simulink model "LoadLevel2_VF"  (R2023b)
settings: Solver=VariableStepAuto  StartTime=0.0  StopTime=250  RelTol=1e-3
undefined symbols (not defined in the file): a, Ac, Bc, Cc, D1, Dc, Delta, find_system, Fnom, gcbh, I21_init_imag, I21_init_real, Ibase1, Ibase2, Iw1A_init_mag, Iw1A_init_pha, Iw1B_init_mag, Iw1B_init_pha, Iw1C_init_mag, Iw1C_init_pha, Iw2A_init_mag, Iw2A_init_pha, Iw2B_init_mag, Iw2B_init_pha, Iw2C_init_mag, Iw2C_init_pha, j, kr, ks, Nmax, Pnom, psi, RegulatorDeadBand, RegulatorDelay, RegulatorVref, sps_rtmsupport, Vnom1, Vnom2, w, Z1pu, Z2pu, Ztpu
libraries: spsThreePhaseVIMeasurementLib x15, spsThreePhasePISectionLineLib x14, spsThreePhaseParallelRLCLoadLib x11, spsControlledCurrentSourceLib x6, spsThreePhaseTransformerTwoWindingsLib x5, spsThreePhaseBreakerLib x2, spsExcitationSystemLib x2, spsHydraulicTurbineandGovernorLib x2, spsSynchronousMachinepuStandardLib x2, spsThreePhaseSeriesRLCBranchLib x2, spsGroundLib x2, spsSequenceAnalyzerPhasorLib x1
(part 3 of 3)

== system LoadLevel2_VF/Three-Phase OLTC Regulating Transformer (Phasor Type)2/Voltage regulator/On//Off Delay/OFF Delay/Edge Detector ==
  note: Edge or Slope Detector
  In : Inport
  Constant1 : Constant  Value=model
  Demux : Demux  Outputs=2
      settings: DisplayOption=none
  Logical Operator1 : Logic  Operator=OR
  Memory : Memory  InitialCondition=ic  LinearizeAsDelay=on
  Multiport Switch : MultiPortSwitch  InputSameDT=off
  NEGATIVE Edge : Subsystem  TreatAsAtomicUnit=on
  POSITIVE Edge : Subsystem  TreatAsAtomicUnit=on
  either edge : Constant  Value=[1 1]
  neg. edge : Constant  Value=[0 1]
  pos. edge : Constant  Value=[1 0]
  Out : Outport  VectorParamsAs1DForOutWhenUnconnected=off
  wires:
  Logical Operator1/1 -> Out/1
  NEGATIVE Edge/1(OUT) -> Logical Operator1/2
  POSITIVE Edge/1(OUT) -> Logical Operator1/1
  Memory/1 -> POSITIVE Edge/2(IN previous), NEGATIVE Edge/2(IN previous)
  In/1 -> POSITIVE Edge/1(IN), NEGATIVE Edge/1(IN), Memory/1
  pos. edge/1 -> Multiport Switch/2
  neg. edge/1 -> Multiport Switch/3
  Constant1/1 -> Multiport Switch/1
  Multiport Switch/1 -> Demux/1
  Demux/1 -> POSITIVE Edge/Enable
  Demux/2 -> NEGATIVE Edge/Enable
  either edge/1 -> Multiport Switch/4

== system LoadLevel2_VF/Three-Phase OLTC Regulating Transformer (Phasor Type)2/Voltage regulator/On//Off Delay/OFF Delay/Sample & Hold ==
  note: Silvano Casoria
      | Power System Simulation Laboratory
      | IREQ, Hydro-Quebc
  note: Sample and Hold
  In : Inport
  S : Inport  Port=2
  IC=ic : Memory  InitialCondition=ic  InheritSampleTime=on
  Switch : Switch  Threshold=0.5
  "   " : Outport  InitialOutput=0  VectorParamsAs1DForOutWhenUnconnected=off
  wires:
  S/1 -> Switch/2
  In/1 -> Switch/1
  IC=ic/1 -> Switch/3
  Switch/1 -> IC=ic/1, "   "/1

== system LoadLevel2_VF/Three-Phase OLTC Regulating Transformer (Phasor Type)2/Voltage regulator/On//Off Delay/ON Delay/Edge Detector ==
  note: Edge or Slope Detector
  In : Inport
  Constant1 : Constant  Value=model
  Demux : Demux  Outputs=2
      settings: DisplayOption=none
  Logical Operator1 : Logic  Operator=OR
  Memory : Memory  InitialCondition=ic  LinearizeAsDelay=on
  Multiport Switch : MultiPortSwitch  InputSameDT=off
  NEGATIVE Edge : Subsystem  TreatAsAtomicUnit=on
  POSITIVE Edge : Subsystem  TreatAsAtomicUnit=on
  either edge : Constant  Value=[1 1]
  neg. edge : Constant  Value=[0 1]
  pos. edge : Constant  Value=[1 0]
  Out : Outport  VectorParamsAs1DForOutWhenUnconnected=off
  wires:
  Logical Operator1/1 -> Out/1
  NEGATIVE Edge/1(OUT) -> Logical Operator1/2
  POSITIVE Edge/1(OUT) -> Logical Operator1/1
  Memory/1 -> POSITIVE Edge/2(IN previous), NEGATIVE Edge/2(IN previous)
  In/1 -> POSITIVE Edge/1(IN), NEGATIVE Edge/1(IN), Memory/1
  pos. edge/1 -> Multiport Switch/2
  neg. edge/1 -> Multiport Switch/3
  Constant1/1 -> Multiport Switch/1
  Multiport Switch/1 -> Demux/1
  Demux/1 -> POSITIVE Edge/Enable
  Demux/2 -> NEGATIVE Edge/Enable
  either edge/1 -> Multiport Switch/4

== system LoadLevel2_VF/Three-Phase OLTC Regulating Transformer (Phasor Type)2/Voltage regulator/On//Off Delay/ON Delay/Sample & Hold ==
  note: Silvano Casoria
      | Power System Simulation Laboratory
      | IREQ, Hydro-Quebc
  note: Sample and Hold
  In : Inport
  S : Inport  Port=2
  IC=ic : Memory  InitialCondition=ic  InheritSampleTime=on
  Switch : Switch  Threshold=0.5
  "   " : Outport  InitialOutput=0  VectorParamsAs1DForOutWhenUnconnected=off
  wires:
  S/1 -> Switch/2
  In/1 -> Switch/1
  IC=ic/1 -> Switch/3
  Switch/1 -> IC=ic/1, "   "/1

== system LoadLevel2_VF/Three-Phase OLTC Regulating Transformer (Phasor Type)2/Voltage regulator/On//Off Delay1/OFF Delay/Edge Detector ==
  note: Edge or Slope Detector
  In : Inport
  Constant1 : Constant  Value=model
  Demux : Demux  Outputs=2
      settings: DisplayOption=none
  Logical Operator1 : Logic  Operator=OR
  Memory : Memory  InitialCondition=ic  LinearizeAsDelay=on
  Multiport Switch : MultiPortSwitch  InputSameDT=off
  NEGATIVE Edge : Subsystem  TreatAsAtomicUnit=on
  POSITIVE Edge : Subsystem  TreatAsAtomicUnit=on
  either edge : Constant  Value=[1 1]
  neg. edge : Constant  Value=[0 1]
  pos. edge : Constant  Value=[1 0]
  Out : Outport  VectorParamsAs1DForOutWhenUnconnected=off
  wires:
  Logical Operator1/1 -> Out/1
  NEGATIVE Edge/1(OUT) -> Logical Operator1/2
  POSITIVE Edge/1(OUT) -> Logical Operator1/1
  Memory/1 -> POSITIVE Edge/2(IN previous), NEGATIVE Edge/2(IN previous)
  In/1 -> POSITIVE Edge/1(IN), NEGATIVE Edge/1(IN), Memory/1
  pos. edge/1 -> Multiport Switch/2
  neg. edge/1 -> Multiport Switch/3
  Constant1/1 -> Multiport Switch/1
  Multiport Switch/1 -> Demux/1
  Demux/1 -> POSITIVE Edge/Enable
  Demux/2 -> NEGATIVE Edge/Enable
  either edge/1 -> Multiport Switch/4

== system LoadLevel2_VF/Three-Phase OLTC Regulating Transformer (Phasor Type)2/Voltage regulator/On//Off Delay1/OFF Delay/Sample & Hold ==
  note: Silvano Casoria
      | Power System Simulation Laboratory
      | IREQ, Hydro-Quebc
  note: Sample and Hold
  In : Inport
  S : Inport  Port=2
  IC=ic : Memory  InitialCondition=ic  InheritSampleTime=on
  Switch : Switch  Threshold=0.5
  "   " : Outport  InitialOutput=0  VectorParamsAs1DForOutWhenUnconnected=off
  wires:
  S/1 -> Switch/2
  In/1 -> Switch/1
  IC=ic/1 -> Switch/3
  Switch/1 -> IC=ic/1, "   "/1

== system LoadLevel2_VF/Three-Phase OLTC Regulating Transformer (Phasor Type)2/Voltage regulator/On//Off Delay1/ON Delay/Edge Detector ==
  note: Edge or Slope Detector
  In : Inport
  Constant1 : Constant  Value=model
  Demux : Demux  Outputs=2
      settings: DisplayOption=none
  Logical Operator1 : Logic  Operator=OR
  Memory : Memory  InitialCondition=ic  LinearizeAsDelay=on
  Multiport Switch : MultiPortSwitch  InputSameDT=off
  NEGATIVE Edge : Subsystem  TreatAsAtomicUnit=on
  POSITIVE Edge : Subsystem  TreatAsAtomicUnit=on
  either edge : Constant  Value=[1 1]
  neg. edge : Constant  Value=[0 1]
  pos. edge : Constant  Value=[1 0]
  Out : Outport  VectorParamsAs1DForOutWhenUnconnected=off
  wires:
  Logical Operator1/1 -> Out/1
  NEGATIVE Edge/1(OUT) -> Logical Operator1/2
  POSITIVE Edge/1(OUT) -> Logical Operator1/1
  Memory/1 -> POSITIVE Edge/2(IN previous), NEGATIVE Edge/2(IN previous)
  In/1 -> POSITIVE Edge/1(IN), NEGATIVE Edge/1(IN), Memory/1
  pos. edge/1 -> Multiport Switch/2
  neg. edge/1 -> Multiport Switch/3
  Constant1/1 -> Multiport Switch/1
  Multiport Switch/1 -> Demux/1
  Demux/1 -> POSITIVE Edge/Enable
  Demux/2 -> NEGATIVE Edge/Enable
  either edge/1 -> Multiport Switch/4

== system LoadLevel2_VF/Three-Phase OLTC Regulating Transformer (Phasor Type)2/Voltage regulator/On//Off Delay1/ON Delay/Sample & Hold ==
  note: Silvano Casoria
      | Power System Simulation Laboratory
      | IREQ, Hydro-Quebc
  note: Sample and Hold
  In : Inport
  S : Inport  Port=2
  IC=ic : Memory  InitialCondition=ic  InheritSampleTime=on
  Switch : Switch  Threshold=0.5
  "   " : Outport  InitialOutput=0  VectorParamsAs1DForOutWhenUnconnected=off
  wires:
  S/1 -> Switch/2
  In/1 -> Switch/1
  IC=ic/1 -> Switch/3
  Switch/1 -> IC=ic/1, "   "/1

== system LoadLevel2_VF/Three-Phase OLTC Regulating Transformer (Phasor Type)2/Voltage regulator/On//Off Delay/OFF Delay/Edge Detector/NEGATIVE Edge ==
  IN : Inport
  IN previous : Inport  Port=2
  Enable : EnablePort  PropagateVarSize=During execution
  Relational Operator1 : RelationalOperator  Operator=>
  OUT : Outport  VectorParamsAs1DForOutWhenUnconnected=off
  wires:
  Relational Operator1/1 -> OUT/1
  IN previous/1 -> Relational Operator1/1
  IN/1 -> Relational Operator1/2

== system LoadLevel2_VF/Three-Phase OLTC Regulating Transformer (Phasor Type)2/Voltage regulator/On//Off Delay/OFF Delay/Edge Detector/POSITIVE Edge ==
  IN : Inport
  IN previous : Inport  Port=2
  Enable : EnablePort  PropagateVarSize=During execution
  Relational Operator1 : RelationalOperator  Operator=>
  OUT : Outport  VectorParamsAs1DForOutWhenUnconnected=off
  wires:
  Relational Operator1/1 -> OUT/1
  IN previous/1 -> Relational Operator1/2
  IN/1 -> Relational Operator1/1

== system LoadLevel2_VF/Three-Phase OLTC Regulating Transformer (Phasor Type)2/Voltage regulator/On//Off Delay/ON Delay/Edge Detector/NEGATIVE Edge ==
  IN : Inport
  IN previous : Inport  Port=2
  Enable : EnablePort  PropagateVarSize=During execution
  Relational Operator1 : RelationalOperator  Operator=>
  OUT : Outport  VectorParamsAs1DForOutWhenUnconnected=off
  wires:
  Relational Operator1/1 -> OUT/1
  IN previous/1 -> Relational Operator1/1
  IN/1 -> Relational Operator1/2

== system LoadLevel2_VF/Three-Phase OLTC Regulating Transformer (Phasor Type)2/Voltage regulator/On//Off Delay/ON Delay/Edge Detector/POSITIVE Edge ==
  IN : Inport
  IN previous : Inport  Port=2
  Enable : EnablePort  PropagateVarSize=During execution
  Relational Operator1 : RelationalOperator  Operator=>
  OUT : Outport  VectorParamsAs1DForOutWhenUnconnected=off
  wires:
  Relational Operator1/1 -> OUT/1
  IN previous/1 -> Relational Operator1/2
  IN/1 -> Relational Operator1/1

== system LoadLevel2_VF/Three-Phase OLTC Regulating Transformer (Phasor Type)2/Voltage regulator/On//Off Delay1/OFF Delay/Edge Detector/NEGATIVE Edge ==
  IN : Inport
  IN previous : Inport  Port=2
  Enable : EnablePort  PropagateVarSize=During execution
  Relational Operator1 : RelationalOperator  Operator=>
  OUT : Outport  VectorParamsAs1DForOutWhenUnconnected=off
  wires:
  Relational Operator1/1 -> OUT/1
  IN previous/1 -> Relational Operator1/1
  IN/1 -> Relational Operator1/2

== system LoadLevel2_VF/Three-Phase OLTC Regulating Transformer (Phasor Type)2/Voltage regulator/On//Off Delay1/OFF Delay/Edge Detector/POSITIVE Edge ==
  IN : Inport
  IN previous : Inport  Port=2
  Enable : EnablePort  PropagateVarSize=During execution
  Relational Operator1 : RelationalOperator  Operator=>
  OUT : Outport  VectorParamsAs1DForOutWhenUnconnected=off
  wires:
  Relational Operator1/1 -> OUT/1
  IN previous/1 -> Relational Operator1/2
  IN/1 -> Relational Operator1/1

== system LoadLevel2_VF/Three-Phase OLTC Regulating Transformer (Phasor Type)2/Voltage regulator/On//Off Delay1/ON Delay/Edge Detector/NEGATIVE Edge ==
  IN : Inport
  IN previous : Inport  Port=2
  Enable : EnablePort  PropagateVarSize=During execution
  Relational Operator1 : RelationalOperator  Operator=>
  OUT : Outport  VectorParamsAs1DForOutWhenUnconnected=off
  wires:
  Relational Operator1/1 -> OUT/1
  IN previous/1 -> Relational Operator1/1
  IN/1 -> Relational Operator1/2

== system LoadLevel2_VF/Three-Phase OLTC Regulating Transformer (Phasor Type)2/Voltage regulator/On//Off Delay1/ON Delay/Edge Detector/POSITIVE Edge ==
  IN : Inport
  IN previous : Inport  Port=2
  Enable : EnablePort  PropagateVarSize=During execution
  Relational Operator1 : RelationalOperator  Operator=>
  OUT : Outport  VectorParamsAs1DForOutWhenUnconnected=off
  wires:
  Relational Operator1/1 -> OUT/1
  IN previous/1 -> Relational Operator1/2
  IN/1 -> Relational Operator1/1

== matlab function LoadLevel2_VF/Subsystem5/MATLAB Function ==
  data: u input; y output
function y = fcn(u)
if u>0 
    y = u;
else 
    y=0;
end
